simulink model "new_three_axle_vehicle_2dof_3dof_Trucksim"  (R2024b)
settings: Solver=VariableStepAuto  StartTime=0.0  StopTime=20  RelTol=1e-3
libraries: Solver_SF x1
settings Model: Creator=Administrator  LastModifiedBy=ccc
settings DebuggingCC: UnconnectedInputMsg=warning  UnconnectedOutputMsg=warning  UnconnectedLineMsg=warning
settings ModelReferenceCC: EnableRefExpFcnMdlSchedulingChecks=on
settings RTWCC: GPUComputeCapability=3.5  DLArmComputeVersion=19.05

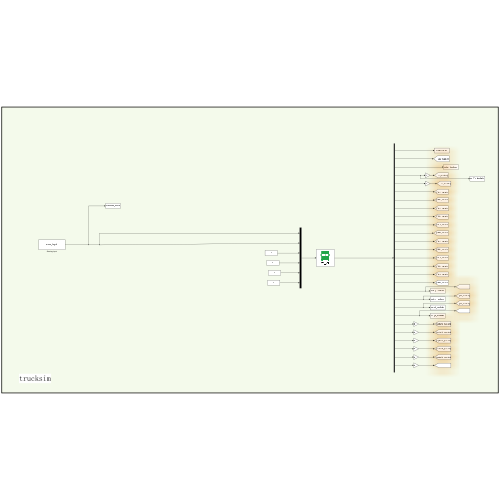
[thumbnail: Simulink's stored preview of the top-level diagram]
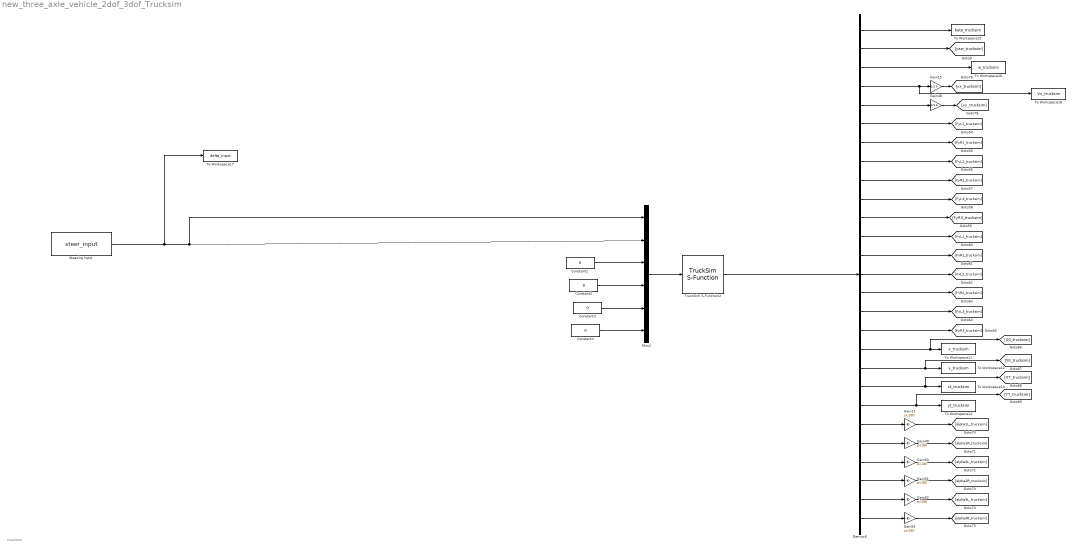
== system new_three_axle_vehicle_2dof_3dof_Trucksim ==
  note: trucksim
  Constant{1..4} (4 alike) : Constant  Value=0
  Demux6 : Demux  Outputs=27
  Gain15 : Gain  Gain=1/3.6
  Gain{17,49..53} (6 alike) : Gain  Gain=pi/180
  Gain48 : Gain  Gain=1/3.6
  Mux2 : Mux  Inputs=6
  Steering Input : FromWorkspace  VariableName=steer_input
  To Workspace11 : ToWorkspace  VariableName=x_trucksim  SaveFormat=Timeseries  SampleTime=-1
  To Workspace12 : ToWorkspace  VariableName=y_trucksim  SaveFormat=Timeseries  SampleTime=-1
  To Workspace13 : ToWorkspace  VariableName=xt_trucksim  SaveFormat=Timeseries  SampleTime=-1
  To Workspace14 : ToWorkspace  VariableName=yt_trucksim  SaveFormat=Timeseries  SampleTime=-1
  To Workspace15 : ToWorkspace  VariableName=beta_trucksim  SaveFormat=Timeseries  SampleTime=-1
  To Workspace16 : ToWorkspace  VariableName=w_trucksim  SaveFormat=Timeseries  SampleTime=-1
  To Workspace17 : ToWorkspace  VariableName=delta_input  SaveFormat=Timeseries  SampleTime=-1
  To Workspace18 : ToWorkspace  VariableName=Vx_trucksim  SaveFormat=Timeseries  SampleTime=-1
  TruckSim S-Function2 : Solver_SF/TruckSim S-Function  Priority=1  SIMFILE=C:\Trucksim2019\TruckSim2019.0_Data\simfile_phase1.sim
      settings: SourceProductName=TruckSim S-Function
  wires:
  Demux6/20 -> [XT_trucksim], To Workspace13/1
  Demux6/3 -> To Workspace16/1
  Demux6/26 -> Gain52/1
  Demux6/23 -> Gain49/1
  Mux2/1 -> TruckSim S-Function2/1
  Demux6/17 -> [FxR3_trucksim]
  Gain15/1 -> [vx_trucksim]
  Gain51/1 -> [alpha2R_trucksim]
  Gain49/1 -> [alpha1R_trucksim]
  Demux6/12 -> [FxL1_trucksim]
  Gain17/1 -> [alpha1L_trucksim]
  Demux6/8 -> [FyL2_trucksim]
  Demux6/11 -> [FyR3_trucksim]
  Demux6/15 -> [FxR2_trucksim]
  Demux6/10 -> [FyL3_trucksim]
  Gain52/1 -> [alpha3L_trucksim]
  Demux6/27 -> Gain53/1
  Demux6/2 -> [yaw_trucksim]
  Gain48/1 -> [vy_trucksim]
  Demux6/18 -> [X0_trucksim], To Workspace11/1
  Demux6/5 -> Gain48/1
  Demux6/24 -> Gain50/1
  Demux6/21 -> [YT_trucksim], To Workspace14/1
  Gain53/1 -> [alpha3R_trucksim]
  Demux6/1 -> To Workspace15/1
  Demux6/19 -> [Y0_trucksim], To Workspace12/1
  Demux6/4 -> To Workspace18/1, Gain15/1
  Demux6/9 -> [FyR2_trucksim]
  Gain50/1 -> [alpha2L_trucksim]
  Demux6/14 -> [FxL2_trucksim]
  Demux6/7 -> [FyR1_trucksim]
  Demux6/25 -> Gain51/1
  Demux6/22 -> Gain17/1
  Demux6/16 -> [FxL3_trucksim]
  TruckSim S-Function2/1 -> Demux6/1
  Demux6/13 -> [FxR1_trucksim]
  Demux6/6 -> [FyL1_trucksim]
  Steering Input/1 -> To Workspace17/1, Mux2/1, Mux2/2
  Constant1/1 -> Mux2/3
  Constant2/1 -> Mux2/4
  Constant3/1 -> Mux2/5
  Constant4/1 -> Mux2/6
